simulink model "subsystem"  (R2020b)
settings: Solver=VariableStepAuto  StartTime=0.0  StopTime=10.0  RelTol=1e-3
settings Model: Creator=Shivani  LastModifiedBy=Shivani

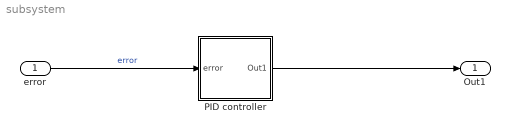
== system subsystem ==
  error : Inport  OutDataTypeStr=double  PortDimensions=1  SampleTime=0
  PID controller : Subsystem  TreatAsAtomicUnit=on
  Out1 : Outport  OutDataTypeStr=double  PortDimensions=1  SampleTime=0
  wires:
  PID controller/1(Out1) -> Out1/1
  error/1 -> PID controller/1(error)  "error"

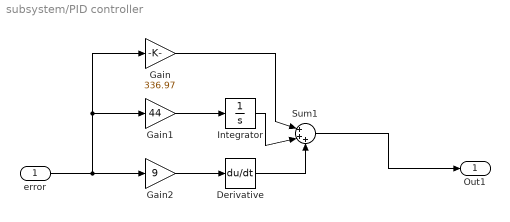
== system subsystem/PID controller ==
  error : Inport
  Derivative : Derivative
  Gain : Gain  Gain=336.97
  Gain1 : Gain  Gain=44
  Gain2 : Gain  Gain=9
  Integrator : Integrator
  Sum1 : Sum  Inputs=|+++
  Out1 : Outport
  wires:
  Gain1/1 -> Integrator/1
  Gain/1 -> Sum1/1
  Sum1/1 -> Out1/1
  error/1 -> Gain2/1, Gain1/1, Gain/1
  Derivative/1 -> Sum1/3
  Gain2/1 -> Derivative/1
  Integrator/1 -> Sum1/2
